simulink model "Robot"  (R2022b)
settings: Solver=FixedStepDiscrete  StartTime=0.0  StopTime=30  FixedStep=0.001  RelTol=1e-3
InitFcn:
  | load("BusConfig.mat");
undefined symbols (not defined in the file or in its folder): DiscIntNeverNeededParam
libraries: slrealtimeethercatlib x119, simulink x20
(part 5 of 7)

== system Robot/Motor1 Torque Control Init Frame/Set MasterState to OP Frame/If Action Subsystem7 ==
  In1 : Inport
  Action Port : ActionPort  ActionPortLabel=if((u1 == 8))
  Discrete-Time Integrator : DiscreteIntegrator  SampleTime=-1  ICPrevOutput=DiscIntNeverNeededParam  ICPrevScaledInput=DiscIntNeverNeededParam
  Out1 : Outport
  wires:
  In1/1 -> Discrete-Time Integrator/1
  Discrete-Time Integrator/1 -> Out1/1

== system Robot/Motor1 Torque Control Init Frame/Set MasterState to SafeOP Frame/If Action Subsystem5 ==
  In1 : Inport
  Action Port : ActionPort  ActionPortLabel=if((u1 > 0.1))
  Out1 : Outport
  wires:
  In1/1 -> Out1/1

== system Robot/Motor1 Torque Control Init Frame/Set MasterState to SafeOP Frame/If Action Subsystem6 ==
  In1 : Inport
  Action Port : ActionPort  ActionPortLabel=else
  Out1 : Outport
  wires:
  In1/1 -> Out1/1

== system Robot/Motor1 Torque Control Init Frame/Set MasterState to SafeOP Frame/If Action Subsystem7 ==
  In1 : Inport
  Action Port : ActionPort  ActionPortLabel=if((u1 == 4))
  Discrete-Time Integrator : DiscreteIntegrator  SampleTime=-1  ICPrevOutput=DiscIntNeverNeededParam  ICPrevScaledInput=DiscIntNeverNeededParam
  Out1 : Outport
  wires:
  In1/1 -> Discrete-Time Integrator/1
  Discrete-Time Integrator/1 -> Out1/1

== system Robot/Motor1 Torque Control Init Frame/State_10_Enable/Subsystem ==
  Case : Inport
  Case Default : Inport  Port=2
  Constant : Constant
  Constant1 : Constant  Value=0
  Constant2 : Constant  Value=TaskIndex
  Merge : Merge
  Switch Case Action Subsystem : Subsystem  TreatAsAtomicUnit=on
  Switch Case Action Subsystem1 : Subsystem  TreatAsAtomicUnit=on
  Enable : Outport
  FinishIndex : Outport  Port=2
  wires:
  Constant/1 -> Switch Case Action Subsystem/1(In1)
  Case/1 -> Switch Case Action Subsystem/Action
  Switch Case Action Subsystem/1(Out1) -> Merge/1
  Merge/1 -> Enable/1
  Case Default/1 -> Switch Case Action Subsystem1/Action
  Constant1/1 -> Switch Case Action Subsystem1/1(In1)
  Switch Case Action Subsystem1/1(Default) -> Merge/2
  Constant2/1 -> FinishIndex/1

== system Robot/Motor1 Torque Control Init Frame/State_11_Enable/Subsystem ==
  Case : Inport
  Case Default : Inport  Port=2
  Constant : Constant
  Constant1 : Constant  Value=0
  Constant2 : Constant  Value=TaskIndex
  Merge : Merge
  Switch Case Action Subsystem : Subsystem  TreatAsAtomicUnit=on
  Switch Case Action Subsystem1 : Subsystem  TreatAsAtomicUnit=on
  Enable : Outport
  FinishIndex : Outport  Port=2
  wires:
  Constant/1 -> Switch Case Action Subsystem/1(In1)
  Case/1 -> Switch Case Action Subsystem/Action
  Switch Case Action Subsystem/1(Out1) -> Merge/1
  Merge/1 -> Enable/1
  Case Default/1 -> Switch Case Action Subsystem1/Action
  Constant1/1 -> Switch Case Action Subsystem1/1(In1)
  Switch Case Action Subsystem1/1(Default) -> Merge/2
  Constant2/1 -> FinishIndex/1

== system Robot/Motor1 Torque Control Init Frame/State_12_Enable/Subsystem ==
  Case : Inport
  Case Default : Inport  Port=2
  Constant : Constant
  Constant1 : Constant  Value=0
  Constant2 : Constant  Value=TaskIndex
  Merge : Merge
  Switch Case Action Subsystem : Subsystem  TreatAsAtomicUnit=on
  Switch Case Action Subsystem1 : Subsystem  TreatAsAtomicUnit=on
  Enable : Outport
  FinishIndex : Outport  Port=2
  wires:
  Constant/1 -> Switch Case Action Subsystem/1(In1)
  Case/1 -> Switch Case Action Subsystem/Action
  Switch Case Action Subsystem/1(Out1) -> Merge/1
  Merge/1 -> Enable/1
  Case Default/1 -> Switch Case Action Subsystem1/Action
  Constant1/1 -> Switch Case Action Subsystem1/1(In1)
  Switch Case Action Subsystem1/1(Default) -> Merge/2
  Constant2/1 -> FinishIndex/1

== system Robot/Motor1 Torque Control Init Frame/State_13_Enable/Subsystem ==
  Case : Inport
  Case Default : Inport  Port=2
  Constant : Constant
  Constant1 : Constant  Value=0
  Constant2 : Constant  Value=TaskIndex
  Merge : Merge
  Switch Case Action Subsystem : Subsystem  TreatAsAtomicUnit=on
  Switch Case Action Subsystem1 : Subsystem  TreatAsAtomicUnit=on
  Enable : Outport
  FinishIndex : Outport  Port=2
  wires:
  Constant/1 -> Switch Case Action Subsystem/1(In1)
  Case/1 -> Switch Case Action Subsystem/Action
  Switch Case Action Subsystem/1(Out1) -> Merge/1
  Merge/1 -> Enable/1
  Case Default/1 -> Switch Case Action Subsystem1/Action
  Constant1/1 -> Switch Case Action Subsystem1/1(In1)
  Switch Case Action Subsystem1/1(Default) -> Merge/2
  Constant2/1 -> FinishIndex/1

== system Robot/Motor1 Torque Control Init Frame/State_1_Enable/Subsystem ==
  Case : Inport
  Case Default : Inport  Port=2
  Constant : Constant
  Constant1 : Constant  Value=0
  Constant2 : Constant  Value=TaskIndex
  Merge : Merge
  Switch Case Action Subsystem : Subsystem  TreatAsAtomicUnit=on
  Switch Case Action Subsystem1 : Subsystem  TreatAsAtomicUnit=on
  Enable : Outport
  FinishIndex : Outport  Port=2
  wires:
  Constant/1 -> Switch Case Action Subsystem/1(In1)
  Case/1 -> Switch Case Action Subsystem/Action
  Switch Case Action Subsystem/1(Out1) -> Merge/1
  Merge/1 -> Enable/1
  Case Default/1 -> Switch Case Action Subsystem1/Action
  Constant1/1 -> Switch Case Action Subsystem1/1(In1)
  Switch Case Action Subsystem1/1(Default) -> Merge/2
  Constant2/1 -> FinishIndex/1

== system Robot/Motor1 Torque Control Init Frame/State_2_Enable/Subsystem ==
  Case : Inport
  Case Default : Inport  Port=2
  Constant : Constant
  Constant1 : Constant  Value=0
  Constant2 : Constant  Value=TaskIndex
  Merge : Merge
  Switch Case Action Subsystem : Subsystem  TreatAsAtomicUnit=on
  Switch Case Action Subsystem1 : Subsystem  TreatAsAtomicUnit=on
  Enable : Outport
  FinishIndex : Outport  Port=2
  wires:
  Constant/1 -> Switch Case Action Subsystem/1(In1)
  Case/1 -> Switch Case Action Subsystem/Action
  Switch Case Action Subsystem/1(Out1) -> Merge/1
  Merge/1 -> Enable/1
  Case Default/1 -> Switch Case Action Subsystem1/Action
  Constant1/1 -> Switch Case Action Subsystem1/1(In1)
  Switch Case Action Subsystem1/1(Default) -> Merge/2
  Constant2/1 -> FinishIndex/1

== system Robot/Motor1 Torque Control Init Frame/State_3_Enable/Subsystem ==
  Case : Inport
  Case Default : Inport  Port=2
  Constant : Constant
  Constant1 : Constant  Value=0
  Constant2 : Constant  Value=TaskIndex
  Merge : Merge
  Switch Case Action Subsystem : Subsystem  TreatAsAtomicUnit=on
  Switch Case Action Subsystem1 : Subsystem  TreatAsAtomicUnit=on
  Enable : Outport
  FinishIndex : Outport  Port=2
  wires:
  Constant/1 -> Switch Case Action Subsystem/1(In1)
  Case/1 -> Switch Case Action Subsystem/Action
  Switch Case Action Subsystem/1(Out1) -> Merge/1
  Merge/1 -> Enable/1
  Case Default/1 -> Switch Case Action Subsystem1/Action
  Constant1/1 -> Switch Case Action Subsystem1/1(In1)
  Switch Case Action Subsystem1/1(Default) -> Merge/2
  Constant2/1 -> FinishIndex/1

== system Robot/Motor1 Torque Control Init Frame/State_4_Enable/Subsystem ==
  Case : Inport
  Case Default : Inport  Port=2
  Constant : Constant
  Constant1 : Constant  Value=0
  Constant2 : Constant  Value=TaskIndex
  Merge : Merge
  Switch Case Action Subsystem : Subsystem  TreatAsAtomicUnit=on
  Switch Case Action Subsystem1 : Subsystem  TreatAsAtomicUnit=on
  Enable : Outport
  FinishIndex : Outport  Port=2
  wires:
  Constant/1 -> Switch Case Action Subsystem/1(In1)
  Case/1 -> Switch Case Action Subsystem/Action
  Switch Case Action Subsystem/1(Out1) -> Merge/1
  Merge/1 -> Enable/1
  Case Default/1 -> Switch Case Action Subsystem1/Action
  Constant1/1 -> Switch Case Action Subsystem1/1(In1)
  Switch Case Action Subsystem1/1(Default) -> Merge/2
  Constant2/1 -> FinishIndex/1

== system Robot/Motor1 Torque Control Init Frame/State_5_Enable/Subsystem ==
  Case : Inport
  Case Default : Inport  Port=2
  Constant : Constant
  Constant1 : Constant  Value=0
  Constant2 : Constant  Value=TaskIndex
  Merge : Merge
  Switch Case Action Subsystem : Subsystem  TreatAsAtomicUnit=on
  Switch Case Action Subsystem1 : Subsystem  TreatAsAtomicUnit=on
  Enable : Outport
  FinishIndex : Outport  Port=2
  wires:
  Constant/1 -> Switch Case Action Subsystem/1(In1)
  Case/1 -> Switch Case Action Subsystem/Action
  Switch Case Action Subsystem/1(Out1) -> Merge/1
  Merge/1 -> Enable/1
  Case Default/1 -> Switch Case Action Subsystem1/Action
  Constant1/1 -> Switch Case Action Subsystem1/1(In1)
  Switch Case Action Subsystem1/1(Default) -> Merge/2
  Constant2/1 -> FinishIndex/1

== system Robot/Motor1 Torque Control Init Frame/State_6_Enable/Subsystem ==
  Case : Inport
  Case Default : Inport  Port=2
  Constant : Constant
  Constant1 : Constant  Value=0
  Constant2 : Constant  Value=TaskIndex
  Merge : Merge
  Switch Case Action Subsystem : Subsystem  TreatAsAtomicUnit=on
  Switch Case Action Subsystem1 : Subsystem  TreatAsAtomicUnit=on
  Enable : Outport
  FinishIndex : Outport  Port=2
  wires:
  Constant/1 -> Switch Case Action Subsystem/1(In1)
  Case/1 -> Switch Case Action Subsystem/Action
  Switch Case Action Subsystem/1(Out1) -> Merge/1
  Merge/1 -> Enable/1
  Case Default/1 -> Switch Case Action Subsystem1/Action
  Constant1/1 -> Switch Case Action Subsystem1/1(In1)
  Switch Case Action Subsystem1/1(Default) -> Merge/2
  Constant2/1 -> FinishIndex/1

== system Robot/Motor1 Torque Control Init Frame/State_7_Enable/Subsystem ==
  Case : Inport
  Case Default : Inport  Port=2
  Constant : Constant
  Constant1 : Constant  Value=0
  Constant2 : Constant  Value=TaskIndex
  Merge : Merge
  Switch Case Action Subsystem : Subsystem  TreatAsAtomicUnit=on
  Switch Case Action Subsystem1 : Subsystem  TreatAsAtomicUnit=on
  Enable : Outport
  FinishIndex : Outport  Port=2
  wires:
  Constant/1 -> Switch Case Action Subsystem/1(In1)
  Case/1 -> Switch Case Action Subsystem/Action
  Switch Case Action Subsystem/1(Out1) -> Merge/1
  Merge/1 -> Enable/1
  Case Default/1 -> Switch Case Action Subsystem1/Action
  Constant1/1 -> Switch Case Action Subsystem1/1(In1)
  Switch Case Action Subsystem1/1(Default) -> Merge/2
  Constant2/1 -> FinishIndex/1

== system Robot/Motor1 Torque Control Init Frame/State_8_Enable/Subsystem ==
  Case : Inport
  Case Default : Inport  Port=2
  Constant : Constant
  Constant1 : Constant  Value=0
  Constant2 : Constant  Value=TaskIndex
  Merge : Merge
  Switch Case Action Subsystem : Subsystem  TreatAsAtomicUnit=on
  Switch Case Action Subsystem1 : Subsystem  TreatAsAtomicUnit=on
  Enable : Outport
  FinishIndex : Outport  Port=2
  wires:
  Constant/1 -> Switch Case Action Subsystem/1(In1)
  Case/1 -> Switch Case Action Subsystem/Action
  Switch Case Action Subsystem/1(Out1) -> Merge/1
  Merge/1 -> Enable/1
  Case Default/1 -> Switch Case Action Subsystem1/Action
  Constant1/1 -> Switch Case Action Subsystem1/1(In1)
  Switch Case Action Subsystem1/1(Default) -> Merge/2
  Constant2/1 -> FinishIndex/1

== system Robot/Motor1 Torque Control Init Frame/State_9_Enable/Subsystem ==
  Case : Inport
  Case Default : Inport  Port=2
  Constant : Constant
  Constant1 : Constant  Value=0
  Constant2 : Constant  Value=TaskIndex
  Merge : Merge
  Switch Case Action Subsystem : Subsystem  TreatAsAtomicUnit=on
  Switch Case Action Subsystem1 : Subsystem  TreatAsAtomicUnit=on
  Enable : Outport
  FinishIndex : Outport  Port=2
  wires:
  Constant/1 -> Switch Case Action Subsystem/1(In1)
  Case/1 -> Switch Case Action Subsystem/Action
  Switch Case Action Subsystem/1(Out1) -> Merge/1
  Merge/1 -> Enable/1
  Case Default/1 -> Switch Case Action Subsystem1/Action
  Constant1/1 -> Switch Case Action Subsystem1/1(In1)
  Switch Case Action Subsystem1/1(Default) -> Merge/2
  Constant2/1 -> FinishIndex/1

== system Robot/Motor2 Torque Control Init Frame/Get MasterState OP Frame/If Action Subsystem5 ==
  In1 : Inport
  Action Port : ActionPort  ActionPortLabel=if((u1 == 8))
  Out1 : Outport
  wires:
  In1/1 -> Out1/1

== system Robot/Motor2 Torque Control Init Frame/Get MasterState OP Frame/If Action Subsystem6 ==
  In1 : Inport
  Action Port : ActionPort  ActionPortLabel=else
  Out1 : Outport
  wires:
  In1/1 -> Out1/1

== system Robot/Motor2 Torque Control Init Frame/Get MasterState OP Frame/If Action Subsystem7 ==
  In1 : Inport
  Action Port : ActionPort  ActionPortLabel=if((u1 == 4663))
  Discrete-Time Integrator : DiscreteIntegrator  SampleTime=-1  ICPrevOutput=DiscIntNeverNeededParam  ICPrevScaledInput=DiscIntNeverNeededParam
  Out1 : Outport
  wires:
  In1/1 -> Discrete-Time Integrator/1
  Discrete-Time Integrator/1 -> Out1/1

== system Robot/Motor2 Torque Control Init Frame/PDO Set 0x6040:6->7->15 Frame/If Action Subsystem ==
  In1 : Inport
  Action Port : ActionPort  ActionPortLabel=if((u1 == 720)&(u2 == 500))
  Out1 : Outport
  wires:
  In1/1 -> Out1/1

== system Robot/Motor2 Torque Control Init Frame/PDO Set 0x6040:6->7->15 Frame/If Action Subsystem1 ==
  In1 : Inport
  Action Port : ActionPort  ActionPortLabel=elseif((u1 == 689)&(u2 == 500))
  Out1 : Outport
  wires:
  In1/1 -> Out1/1

== system Robot/Motor2 Torque Control Init Frame/PDO Set 0x6040:6->7->15 Frame/If Action Subsystem2 ==
  In1 : Inport
  Action Port : ActionPort  ActionPortLabel=elseif( (u1 == 691)&(u2 == 500))
  Out1 : Outport
  wires:
  In1/1 -> Out1/1

== system Robot/Motor2 Torque Control Init Frame/PDO Set 0x6040:6->7->15 Frame/If Action Subsystem4 ==
  In1 : Inport
  Action Port : ActionPort  ActionPortLabel=else
  Out1 : Outport
  wires:
  In1/1 -> Out1/1

== system Robot/Motor2 Torque Control Init Frame/PDO Set 0x6040:6->7->15 Frame/If Action Subsystem5 ==
  In1 : Inport
  Action Port : ActionPort  ActionPortLabel=if((u1 >= 0.1))
  Out1 : Outport
  wires:
  In1/1 -> Out1/1

== system Robot/Motor2 Torque Control Init Frame/PDO Set 0x6040:6->7->15 Frame/If Action Subsystem6 ==
  In1 : Inport
  Action Port : ActionPort  ActionPortLabel=else
  Out1 : Outport
  wires:
  In1/1 -> Out1/1

== system Robot/Motor2 Torque Control Init Frame/PDO Set 0x6040:6->7->15 Frame/If Action Subsystem7 ==
  In1 : Inport
  Action Port : ActionPort  ActionPortLabel=if((u1 == 4663)|(u1 == 4791))
  Discrete-Time Integrator : DiscreteIntegrator  SampleTime=-1  ICPrevOutput=DiscIntNeverNeededParam  ICPrevScaledInput=DiscIntNeverNeededParam
  Out1 : Outport
  wires:
  In1/1 -> Discrete-Time Integrator/1
  Discrete-Time Integrator/1 -> Out1/1

== system Robot/Motor2 Torque Control Init Frame/SDO Get 0x6075 Frame/If Action Subsystem5 ==
  In1 : Inport
  Action Port : ActionPort  ActionPortLabel=if((u1 == 2))
  Out1 : Outport
  wires:
  In1/1 -> Out1/1

== system Robot/Motor2 Torque Control Init Frame/SDO Get 0x6075 Frame/If Action Subsystem6 ==
  In1 : Inport
  Action Port : ActionPort  ActionPortLabel=else
  Out1 : Outport
  wires:
  In1/1 -> Out1/1

== system Robot/Motor2 Torque Control Init Frame/SDO Get 0x6075 Frame/If Action Subsystem7 ==
  In1 : Inport
  Action Port : ActionPort  ActionPortLabel=if((u1 == 4663))
  Discrete-Time Integrator : DiscreteIntegrator  SampleTime=-1  ICPrevOutput=DiscIntNeverNeededParam  ICPrevScaledInput=DiscIntNeverNeededParam
  Out1 : Outport
  wires:
  In1/1 -> Discrete-Time Integrator/1
  Discrete-Time Integrator/1 -> Out1/1

== system Robot/Motor2 Torque Control Init Frame/SDO Set 0x6040:15 Frame/If Action Subsystem1 ==
  In1 : Inport
  Action Port : ActionPort  ActionPortLabel=if((u1 >= 0.1))
  Out1 : Outport
  wires:
  In1/1 -> Out1/1

== system Robot/Motor2 Torque Control Init Frame/SDO Set 0x6040:15 Frame/If Action Subsystem2 ==
  In1 : Inport
  Action Port : ActionPort  ActionPortLabel=else
  Out1 : Outport
  wires:
  In1/1 -> Out1/1

== system Robot/Motor2 Torque Control Init Frame/SDO Set 0x6040:15 Frame/If Action Subsystem3 ==
  In1 : Inport
  Action Port : ActionPort  ActionPortLabel=if((u1 == u2))
  Discrete-Time Integrator : DiscreteIntegrator  SampleTime=-1  ICPrevOutput=DiscIntNeverNeededParam  ICPrevScaledInput=DiscIntNeverNeededParam
  Out1 : Outport
  wires:
  In1/1 -> Discrete-Time Integrator/1
  Discrete-Time Integrator/1 -> Out1/1

== system Robot/Motor2 Torque Control Init Frame/SDO Set 0x6040:15 Frame/If Action Subsystem5 ==
  In1 : Inport
  Action Port : ActionPort  ActionPortLabel=if((u1 == 2))
  Out1 : Outport
  wires:
  In1/1 -> Out1/1

== system Robot/Motor2 Torque Control Init Frame/SDO Set 0x6040:15 Frame/If Action Subsystem6 ==
  In1 : Inport
  Action Port : ActionPort  ActionPortLabel=else
  Out1 : Outport
  wires:
  In1/1 -> Out1/1

== system Robot/Motor2 Torque Control Init Frame/SDO Set 0x6040:15 Frame/If Action Subsystem7 ==
  In1 : Inport
  Action Port : ActionPort  ActionPortLabel=if((u1 == 4663))
  Discrete-Time Integrator : DiscreteIntegrator  SampleTime=-1  ICPrevOutput=DiscIntNeverNeededParam  ICPrevScaledInput=DiscIntNeverNeededParam
  Out1 : Outport
  wires:
  In1/1 -> Discrete-Time Integrator/1
  Discrete-Time Integrator/1 -> Out1/1

== system Robot/Motor2 Torque Control Init Frame/SDO Set 0x6040:31 Frame/If Action Subsystem1 ==
  In1 : Inport
  Action Port : ActionPort  ActionPortLabel=if((u1 >= 0.1))
  Out1 : Outport
  wires:
  In1/1 -> Out1/1

== system Robot/Motor2 Torque Control Init Frame/SDO Set 0x6040:31 Frame/If Action Subsystem2 ==
  In1 : Inport
  Action Port : ActionPort  ActionPortLabel=else
  Out1 : Outport
  wires:
  In1/1 -> Out1/1

== system Robot/Motor2 Torque Control Init Frame/SDO Set 0x6040:31 Frame/If Action Subsystem3 ==
  In1 : Inport
  Action Port : ActionPort  ActionPortLabel=if((u1 == u2))
  Discrete-Time Integrator : DiscreteIntegrator  SampleTime=-1  ICPrevOutput=DiscIntNeverNeededParam  ICPrevScaledInput=DiscIntNeverNeededParam
  Out1 : Outport
  wires:
  In1/1 -> Discrete-Time Integrator/1
  Discrete-Time Integrator/1 -> Out1/1

== system Robot/Motor2 Torque Control Init Frame/SDO Set 0x6040:31 Frame/If Action Subsystem5 ==
  In1 : Inport
  Action Port : ActionPort  ActionPortLabel=if((u1 == 2))
  Out1 : Outport
  wires:
  In1/1 -> Out1/1

== system Robot/Motor2 Torque Control Init Frame/SDO Set 0x6040:31 Frame/If Action Subsystem6 ==
  In1 : Inport
  Action Port : ActionPort  ActionPortLabel=else
  Out1 : Outport
  wires:
  In1/1 -> Out1/1

== system Robot/Motor2 Torque Control Init Frame/SDO Set 0x6040:31 Frame/If Action Subsystem7 ==
  In1 : Inport
  Action Port : ActionPort  ActionPortLabel=if((u1 == 4663))
  Discrete-Time Integrator : DiscreteIntegrator  SampleTime=-1  ICPrevOutput=DiscIntNeverNeededParam  ICPrevScaledInput=DiscIntNeverNeededParam
  Out1 : Outport
  wires:
  In1/1 -> Discrete-Time Integrator/1
  Discrete-Time Integrator/1 -> Out1/1

== system Robot/Motor2 Torque Control Init Frame/SDO Set 0x6040:6 Frame/If Action Subsystem1 ==
  In1 : Inport
  Action Port : ActionPort  ActionPortLabel=if((u1 >= 0.1))
  Out1 : Outport
  wires:
  In1/1 -> Out1/1

== system Robot/Motor2 Torque Control Init Frame/SDO Set 0x6040:6 Frame/If Action Subsystem2 ==
  In1 : Inport
  Action Port : ActionPort  ActionPortLabel=else
  Out1 : Outport
  wires:
  In1/1 -> Out1/1

== system Robot/Motor2 Torque Control Init Frame/SDO Set 0x6040:6 Frame/If Action Subsystem3 ==
  In1 : Inport
  Action Port : ActionPort  ActionPortLabel=if((u1 == u2))
  Discrete-Time Integrator : DiscreteIntegrator  SampleTime=-1  ICPrevOutput=DiscIntNeverNeededParam  ICPrevScaledInput=DiscIntNeverNeededParam
  Out1 : Outport
  wires:
  In1/1 -> Discrete-Time Integrator/1
  Discrete-Time Integrator/1 -> Out1/1

== system Robot/Motor2 Torque Control Init Frame/SDO Set 0x6040:6 Frame/If Action Subsystem5 ==
  In1 : Inport
  Action Port : ActionPort  ActionPortLabel=if((u1 == 2))
  Out1 : Outport
  wires:
  In1/1 -> Out1/1

== system Robot/Motor2 Torque Control Init Frame/SDO Set 0x6040:6 Frame/If Action Subsystem6 ==
  In1 : Inport
  Action Port : ActionPort  ActionPortLabel=else
  Out1 : Outport
  wires:
  In1/1 -> Out1/1

== system Robot/Motor2 Torque Control Init Frame/SDO Set 0x6040:6 Frame/If Action Subsystem7 ==
  In1 : Inport
  Action Port : ActionPort  ActionPortLabel=if((u1 == 4663))
  Discrete-Time Integrator : DiscreteIntegrator  SampleTime=-1  ICPrevOutput=DiscIntNeverNeededParam  ICPrevScaledInput=DiscIntNeverNeededParam
  Out1 : Outport
  wires:
  In1/1 -> Discrete-Time Integrator/1
  Discrete-Time Integrator/1 -> Out1/1

== system Robot/Motor2 Torque Control Init Frame/SDO Set 0x6040:7 Frame/If Action Subsystem1 ==
  In1 : Inport
  Action Port : ActionPort  ActionPortLabel=if((u1 >= 0.1))
  Out1 : Outport
  wires:
  In1/1 -> Out1/1

== system Robot/Motor2 Torque Control Init Frame/SDO Set 0x6040:7 Frame/If Action Subsystem2 ==
  In1 : Inport
  Action Port : ActionPort  ActionPortLabel=else
  Out1 : Outport
  wires:
  In1/1 -> Out1/1

== system Robot/Motor2 Torque Control Init Frame/SDO Set 0x6040:7 Frame/If Action Subsystem3 ==
  In1 : Inport
  Action Port : ActionPort  ActionPortLabel=if((u1 == u2))
  Discrete-Time Integrator : DiscreteIntegrator  SampleTime=-1  ICPrevOutput=DiscIntNeverNeededParam  ICPrevScaledInput=DiscIntNeverNeededParam
  Out1 : Outport
  wires:
  In1/1 -> Discrete-Time Integrator/1
  Discrete-Time Integrator/1 -> Out1/1

== system Robot/Motor2 Torque Control Init Frame/SDO Set 0x6040:7 Frame/If Action Subsystem5 ==
  In1 : Inport
  Action Port : ActionPort  ActionPortLabel=if((u1 == 2))
  Out1 : Outport
  wires:
  In1/1 -> Out1/1

== system Robot/Motor2 Torque Control Init Frame/SDO Set 0x6040:7 Frame/If Action Subsystem6 ==
  In1 : Inport
  Action Port : ActionPort  ActionPortLabel=else
  Out1 : Outport
  wires:
  In1/1 -> Out1/1

== system Robot/Motor2 Torque Control Init Frame/SDO Set 0x6040:7 Frame/If Action Subsystem7 ==
  In1 : Inport
  Action Port : ActionPort  ActionPortLabel=if((u1 == 4663))
  Discrete-Time Integrator : DiscreteIntegrator  SampleTime=-1  ICPrevOutput=DiscIntNeverNeededParam  ICPrevScaledInput=DiscIntNeverNeededParam
  Out1 : Outport
  wires:
  In1/1 -> Discrete-Time Integrator/1
  Discrete-Time Integrator/1 -> Out1/1

== system Robot/Motor2 Torque Control Init Frame/SDO Set 0x6060:10 Frame/If Action Subsystem5 ==
  In1 : Inport
  Action Port : ActionPort  ActionPortLabel=if((u1 == 2))
  Out1 : Outport
  wires:
  In1/1 -> Out1/1

== system Robot/Motor2 Torque Control Init Frame/SDO Set 0x6060:10 Frame/If Action Subsystem6 ==
  In1 : Inport
  Action Port : ActionPort  ActionPortLabel=else
  Out1 : Outport
  wires:
  In1/1 -> Out1/1

== system Robot/Motor2 Torque Control Init Frame/SDO Set 0x6060:10 Frame/If Action Subsystem7 ==
  In1 : Inport
  Action Port : ActionPort  ActionPortLabel=if((u1 == 4663))
  Discrete-Time Integrator : DiscreteIntegrator  SampleTime=-1  ICPrevOutput=DiscIntNeverNeededParam  ICPrevScaledInput=DiscIntNeverNeededParam
  Out1 : Outport
  wires:
  In1/1 -> Discrete-Time Integrator/1
  Discrete-Time Integrator/1 -> Out1/1

== system Robot/Motor2 Torque Control Init Frame/SDO Set 0x6060:6 Frame/If Action Subsystem5 ==
  In1 : Inport
  Action Port : ActionPort  ActionPortLabel=if((u1 == 2))
  Out1 : Outport
  wires:
  In1/1 -> Out1/1

== system Robot/Motor2 Torque Control Init Frame/SDO Set 0x6060:6 Frame/If Action Subsystem6 ==
  In1 : Inport
  Action Port : ActionPort  ActionPortLabel=else
  Out1 : Outport
  wires:
  In1/1 -> Out1/1

== system Robot/Motor2 Torque Control Init Frame/SDO Set 0x6060:6 Frame/If Action Subsystem7 ==
  In1 : Inport
  Action Port : ActionPort  ActionPortLabel=if((u1 == 4663))
  Discrete-Time Integrator : DiscreteIntegrator  SampleTime=-1  ICPrevOutput=DiscIntNeverNeededParam  ICPrevScaledInput=DiscIntNeverNeededParam
  Out1 : Outport
  wires:
  In1/1 -> Discrete-Time Integrator/1
  Discrete-Time Integrator/1 -> Out1/1

== system Robot/Motor2 Torque Control Init Frame/SDO Set 0x6080:-1 Frame/If Action Subsystem5 ==
  In1 : Inport
  Action Port : ActionPort  ActionPortLabel=if((u1 == 2))
  Out1 : Outport
  wires:
  In1/1 -> Out1/1

== system Robot/Motor2 Torque Control Init Frame/SDO Set 0x6080:-1 Frame/If Action Subsystem6 ==
  In1 : Inport
  Action Port : ActionPort  ActionPortLabel=else
  Out1 : Outport
  wires:
  In1/1 -> Out1/1

== system Robot/Motor2 Torque Control Init Frame/SDO Set 0x6080:-1 Frame/If Action Subsystem7 ==
  In1 : Inport
  Action Port : ActionPort  ActionPortLabel=if((u1 == 4663))
  Discrete-Time Integrator : DiscreteIntegrator  SampleTime=-1  ICPrevOutput=DiscIntNeverNeededParam  ICPrevScaledInput=DiscIntNeverNeededParam
  Out1 : Outport
  wires:
  In1/1 -> Discrete-Time Integrator/1
  Discrete-Time Integrator/1 -> Out1/1

== system Robot/Motor2 Torque Control Init Frame/SDO Set 0x6098:35 Frame/If Action Subsystem5 ==
  In1 : Inport
  Action Port : ActionPort  ActionPortLabel=if((u1 == 2))
  Out1 : Outport
  wires:
  In1/1 -> Out1/1

== system Robot/Motor2 Torque Control Init Frame/SDO Set 0x6098:35 Frame/If Action Subsystem6 ==
  In1 : Inport
  Action Port : ActionPort  ActionPortLabel=else
  Out1 : Outport
  wires:
  In1/1 -> Out1/1

== system Robot/Motor2 Torque Control Init Frame/SDO Set 0x6098:35 Frame/If Action Subsystem7 ==
  In1 : Inport
  Action Port : ActionPort  ActionPortLabel=if((u1 == 4663))
  Discrete-Time Integrator : DiscreteIntegrator  SampleTime=-1  ICPrevOutput=DiscIntNeverNeededParam  ICPrevScaledInput=DiscIntNeverNeededParam
  Out1 : Outport
  wires:
  In1/1 -> Discrete-Time Integrator/1
  Discrete-Time Integrator/1 -> Out1/1

== system Robot/Motor2 Torque Control Init Frame/Set MasterState to OP Frame/If Action Subsystem5 ==
  In1 : Inport
  Action Port : ActionPort  ActionPortLabel=if((u1 > 0.1))
  Out1 : Outport
  wires:
  In1/1 -> Out1/1

== system Robot/Motor2 Torque Control Init Frame/Set MasterState to OP Frame/If Action Subsystem6 ==
  In1 : Inport
  Action Port : ActionPort  ActionPortLabel=else
  Out1 : Outport
  wires:
  In1/1 -> Out1/1

== system Robot/Motor2 Torque Control Init Frame/Set MasterState to OP Frame/If Action Subsystem7 ==
  In1 : Inport
  Action Port : ActionPort  ActionPortLabel=if((u1 == 8))
  Discrete-Time Integrator : DiscreteIntegrator  SampleTime=-1  ICPrevOutput=DiscIntNeverNeededParam  ICPrevScaledInput=DiscIntNeverNeededParam
  Out1 : Outport
  wires:
  In1/1 -> Discrete-Time Integrator/1
  Discrete-Time Integrator/1 -> Out1/1

== system Robot/Motor2 Torque Control Init Frame/Set MasterState to SafeOP Frame/If Action Subsystem5 ==
  In1 : Inport
  Action Port : ActionPort  ActionPortLabel=if((u1 > 0.1))
  Out1 : Outport
  wires:
  In1/1 -> Out1/1

== system Robot/Motor2 Torque Control Init Frame/Set MasterState to SafeOP Frame/If Action Subsystem6 ==
  In1 : Inport
  Action Port : ActionPort  ActionPortLabel=else
  Out1 : Outport
  wires:
  In1/1 -> Out1/1

== system Robot/Motor2 Torque Control Init Frame/Set MasterState to SafeOP Frame/If Action Subsystem7 ==
  In1 : Inport
  Action Port : ActionPort  ActionPortLabel=if((u1 == 4))
  Discrete-Time Integrator : DiscreteIntegrator  SampleTime=-1  ICPrevOutput=DiscIntNeverNeededParam  ICPrevScaledInput=DiscIntNeverNeededParam
  Out1 : Outport
  wires:
  In1/1 -> Discrete-Time Integrator/1
  Discrete-Time Integrator/1 -> Out1/1

== system Robot/Motor2 Torque Control Init Frame/State_10_Enable/Subsystem ==
  Case : Inport
  Case Default : Inport  Port=2
  Constant : Constant
  Constant1 : Constant  Value=0
  Constant2 : Constant  Value=TaskIndex
  Merge : Merge
  Switch Case Action Subsystem : Subsystem  TreatAsAtomicUnit=on
  Switch Case Action Subsystem1 : Subsystem  TreatAsAtomicUnit=on
  Enable : Outport
  FinishIndex : Outport  Port=2
  wires:
  Constant/1 -> Switch Case Action Subsystem/1(In1)
  Case/1 -> Switch Case Action Subsystem/Action
  Switch Case Action Subsystem/1(Out1) -> Merge/1
  Merge/1 -> Enable/1
  Case Default/1 -> Switch Case Action Subsystem1/Action
  Constant1/1 -> Switch Case Action Subsystem1/1(In1)
  Switch Case Action Subsystem1/1(Default) -> Merge/2
  Constant2/1 -> FinishIndex/1

== system Robot/Motor2 Torque Control Init Frame/State_11_Enable/Subsystem ==
  Case : Inport
  Case Default : Inport  Port=2
  Constant : Constant
  Constant1 : Constant  Value=0
  Constant2 : Constant  Value=TaskIndex
  Merge : Merge
  Switch Case Action Subsystem : Subsystem  TreatAsAtomicUnit=on
  Switch Case Action Subsystem1 : Subsystem  TreatAsAtomicUnit=on
  Enable : Outport
  FinishIndex : Outport  Port=2
  wires:
  Constant/1 -> Switch Case Action Subsystem/1(In1)
  Case/1 -> Switch Case Action Subsystem/Action
  Switch Case Action Subsystem/1(Out1) -> Merge/1
  Merge/1 -> Enable/1
  Case Default/1 -> Switch Case Action Subsystem1/Action
  Constant1/1 -> Switch Case Action Subsystem1/1(In1)
  Switch Case Action Subsystem1/1(Default) -> Merge/2
  Constant2/1 -> FinishIndex/1

== system Robot/Motor2 Torque Control Init Frame/State_12_Enable/Subsystem ==
  Case : Inport
  Case Default : Inport  Port=2
  Constant : Constant
  Constant1 : Constant  Value=0
  Constant2 : Constant  Value=TaskIndex
  Merge : Merge
  Switch Case Action Subsystem : Subsystem  TreatAsAtomicUnit=on
  Switch Case Action Subsystem1 : Subsystem  TreatAsAtomicUnit=on
  Enable : Outport
  FinishIndex : Outport  Port=2
  wires:
  Constant/1 -> Switch Case Action Subsystem/1(In1)
  Case/1 -> Switch Case Action Subsystem/Action
  Switch Case Action Subsystem/1(Out1) -> Merge/1
  Merge/1 -> Enable/1
  Case Default/1 -> Switch Case Action Subsystem1/Action
  Constant1/1 -> Switch Case Action Subsystem1/1(In1)
  Switch Case Action Subsystem1/1(Default) -> Merge/2
  Constant2/1 -> FinishIndex/1

== system Robot/Motor2 Torque Control Init Frame/State_13_Enable/Subsystem ==
  Case : Inport
  Case Default : Inport  Port=2
  Constant : Constant
  Constant1 : Constant  Value=0
  Constant2 : Constant  Value=TaskIndex
  Merge : Merge
  Switch Case Action Subsystem : Subsystem  TreatAsAtomicUnit=on
  Switch Case Action Subsystem1 : Subsystem  TreatAsAtomicUnit=on
  Enable : Outport
  FinishIndex : Outport  Port=2
  wires:
  Constant/1 -> Switch Case Action Subsystem/1(In1)
  Case/1 -> Switch Case Action Subsystem/Action
  Switch Case Action Subsystem/1(Out1) -> Merge/1
  Merge/1 -> Enable/1
  Case Default/1 -> Switch Case Action Subsystem1/Action
  Constant1/1 -> Switch Case Action Subsystem1/1(In1)
  Switch Case Action Subsystem1/1(Default) -> Merge/2
  Constant2/1 -> FinishIndex/1

== system Robot/Motor2 Torque Control Init Frame/State_1_Enable/Subsystem ==
  Case : Inport
  Case Default : Inport  Port=2
  Constant : Constant
  Constant1 : Constant  Value=0
  Constant2 : Constant  Value=TaskIndex
  Merge : Merge
  Switch Case Action Subsystem : Subsystem  TreatAsAtomicUnit=on
  Switch Case Action Subsystem1 : Subsystem  TreatAsAtomicUnit=on
  Enable : Outport
  FinishIndex : Outport  Port=2
  wires:
  Constant/1 -> Switch Case Action Subsystem/1(In1)
  Case/1 -> Switch Case Action Subsystem/Action
  Switch Case Action Subsystem/1(Out1) -> Merge/1
  Merge/1 -> Enable/1
  Case Default/1 -> Switch Case Action Subsystem1/Action
  Constant1/1 -> Switch Case Action Subsystem1/1(In1)
  Switch Case Action Subsystem1/1(Default) -> Merge/2
  Constant2/1 -> FinishIndex/1

== system Robot/Motor2 Torque Control Init Frame/State_2_Enable/Subsystem ==
  Case : Inport
  Case Default : Inport  Port=2
  Constant : Constant
  Constant1 : Constant  Value=0
  Constant2 : Constant  Value=TaskIndex
  Merge : Merge
  Switch Case Action Subsystem : Subsystem  TreatAsAtomicUnit=on
  Switch Case Action Subsystem1 : Subsystem  TreatAsAtomicUnit=on
  Enable : Outport
  FinishIndex : Outport  Port=2
  wires:
  Constant/1 -> Switch Case Action Subsystem/1(In1)
  Case/1 -> Switch Case Action Subsystem/Action
  Switch Case Action Subsystem/1(Out1) -> Merge/1
  Merge/1 -> Enable/1
  Case Default/1 -> Switch Case Action Subsystem1/Action
  Constant1/1 -> Switch Case Action Subsystem1/1(In1)
  Switch Case Action Subsystem1/1(Default) -> Merge/2
  Constant2/1 -> FinishIndex/1

== system Robot/Motor2 Torque Control Init Frame/State_3_Enable/Subsystem ==
  Case : Inport
  Case Default : Inport  Port=2
  Constant : Constant
  Constant1 : Constant  Value=0
  Constant2 : Constant  Value=TaskIndex
  Merge : Merge
  Switch Case Action Subsystem : Subsystem  TreatAsAtomicUnit=on
  Switch Case Action Subsystem1 : Subsystem  TreatAsAtomicUnit=on
  Enable : Outport
  FinishIndex : Outport  Port=2
  wires:
  Constant/1 -> Switch Case Action Subsystem/1(In1)
  Case/1 -> Switch Case Action Subsystem/Action
  Switch Case Action Subsystem/1(Out1) -> Merge/1
  Merge/1 -> Enable/1
  Case Default/1 -> Switch Case Action Subsystem1/Action
  Constant1/1 -> Switch Case Action Subsystem1/1(In1)
  Switch Case Action Subsystem1/1(Default) -> Merge/2
  Constant2/1 -> FinishIndex/1

== system Robot/Motor2 Torque Control Init Frame/State_4_Enable/Subsystem ==
  Case : Inport
  Case Default : Inport  Port=2
  Constant : Constant
  Constant1 : Constant  Value=0
  Constant2 : Constant  Value=TaskIndex
  Merge : Merge
  Switch Case Action Subsystem : Subsystem  TreatAsAtomicUnit=on
  Switch Case Action Subsystem1 : Subsystem  TreatAsAtomicUnit=on
  Enable : Outport
  FinishIndex : Outport  Port=2
  wires:
  Constant/1 -> Switch Case Action Subsystem/1(In1)
  Case/1 -> Switch Case Action Subsystem/Action
  Switch Case Action Subsystem/1(Out1) -> Merge/1
  Merge/1 -> Enable/1
  Case Default/1 -> Switch Case Action Subsystem1/Action
  Constant1/1 -> Switch Case Action Subsystem1/1(In1)
  Switch Case Action Subsystem1/1(Default) -> Merge/2
  Constant2/1 -> FinishIndex/1

== system Robot/Motor2 Torque Control Init Frame/State_5_Enable/Subsystem ==
  Case : Inport
  Case Default : Inport  Port=2
  Constant : Constant
  Constant1 : Constant  Value=0
  Constant2 : Constant  Value=TaskIndex
  Merge : Merge
  Switch Case Action Subsystem : Subsystem  TreatAsAtomicUnit=on
  Switch Case Action Subsystem1 : Subsystem  TreatAsAtomicUnit=on
  Enable : Outport
  FinishIndex : Outport  Port=2
  wires:
  Constant/1 -> Switch Case Action Subsystem/1(In1)
  Case/1 -> Switch Case Action Subsystem/Action
  Switch Case Action Subsystem/1(Out1) -> Merge/1
  Merge/1 -> Enable/1
  Case Default/1 -> Switch Case Action Subsystem1/Action
  Constant1/1 -> Switch Case Action Subsystem1/1(In1)
  Switch Case Action Subsystem1/1(Default) -> Merge/2
  Constant2/1 -> FinishIndex/1

== system Robot/Motor2 Torque Control Init Frame/State_6_Enable/Subsystem ==
  Case : Inport
  Case Default : Inport  Port=2
  Constant : Constant
  Constant1 : Constant  Value=0
  Constant2 : Constant  Value=TaskIndex
  Merge : Merge
  Switch Case Action Subsystem : Subsystem  TreatAsAtomicUnit=on
  Switch Case Action Subsystem1 : Subsystem  TreatAsAtomicUnit=on
  Enable : Outport
  FinishIndex : Outport  Port=2
  wires:
  Constant/1 -> Switch Case Action Subsystem/1(In1)
  Case/1 -> Switch Case Action Subsystem/Action
  Switch Case Action Subsystem/1(Out1) -> Merge/1
  Merge/1 -> Enable/1
  Case Default/1 -> Switch Case Action Subsystem1/Action
  Constant1/1 -> Switch Case Action Subsystem1/1(In1)
  Switch Case Action Subsystem1/1(Default) -> Merge/2
  Constant2/1 -> FinishIndex/1

== system Robot/Motor2 Torque Control Init Frame/State_7_Enable/Subsystem ==
  Case : Inport
  Case Default : Inport  Port=2
  Constant : Constant
  Constant1 : Constant  Value=0
  Constant2 : Constant  Value=TaskIndex
  Merge : Merge
  Switch Case Action Subsystem : Subsystem  TreatAsAtomicUnit=on
  Switch Case Action Subsystem1 : Subsystem  TreatAsAtomicUnit=on
  Enable : Outport
  FinishIndex : Outport  Port=2
  wires:
  Constant/1 -> Switch Case Action Subsystem/1(In1)
  Case/1 -> Switch Case Action Subsystem/Action
  Switch Case Action Subsystem/1(Out1) -> Merge/1
  Merge/1 -> Enable/1
  Case Default/1 -> Switch Case Action Subsystem1/Action
  Constant1/1 -> Switch Case Action Subsystem1/1(In1)
  Switch Case Action Subsystem1/1(Default) -> Merge/2
  Constant2/1 -> FinishIndex/1

== system Robot/Motor2 Torque Control Init Frame/State_8_Enable/Subsystem ==
  Case : Inport
  Case Default : Inport  Port=2
  Constant : Constant
  Constant1 : Constant  Value=0
  Constant2 : Constant  Value=TaskIndex
  Merge : Merge
  Switch Case Action Subsystem : Subsystem  TreatAsAtomicUnit=on
  Switch Case Action Subsystem1 : Subsystem  TreatAsAtomicUnit=on
  Enable : Outport
  FinishIndex : Outport  Port=2
  wires:
  Constant/1 -> Switch Case Action Subsystem/1(In1)
  Case/1 -> Switch Case Action Subsystem/Action
  Switch Case Action Subsystem/1(Out1) -> Merge/1
  Merge/1 -> Enable/1
  Case Default/1 -> Switch Case Action Subsystem1/Action
  Constant1/1 -> Switch Case Action Subsystem1/1(In1)
  Switch Case Action Subsystem1/1(Default) -> Merge/2
  Constant2/1 -> FinishIndex/1

== system Robot/Motor2 Torque Control Init Frame/State_9_Enable/Subsystem ==
  Case : Inport
  Case Default : Inport  Port=2
  Constant : Constant
  Constant1 : Constant  Value=0
  Constant2 : Constant  Value=TaskIndex
  Merge : Merge
  Switch Case Action Subsystem : Subsystem  TreatAsAtomicUnit=on
  Switch Case Action Subsystem1 : Subsystem  TreatAsAtomicUnit=on
  Enable : Outport
  FinishIndex : Outport  Port=2
  wires:
  Constant/1 -> Switch Case Action Subsystem/1(In1)
  Case/1 -> Switch Case Action Subsystem/Action
  Switch Case Action Subsystem/1(Out1) -> Merge/1
  Merge/1 -> Enable/1
  Case Default/1 -> Switch Case Action Subsystem1/Action
  Constant1/1 -> Switch Case Action Subsystem1/1(In1)
  Switch Case Action Subsystem1/1(Default) -> Merge/2
  Constant2/1 -> FinishIndex/1

== system Robot/Motor3 Torque Control Init Frame/Get MasterState OP Frame/If Action Subsystem5 ==
  In1 : Inport
  Action Port : ActionPort  ActionPortLabel=if((u1 == 8))
  Out1 : Outport
  wires:
  In1/1 -> Out1/1

== system Robot/Motor3 Torque Control Init Frame/Get MasterState OP Frame/If Action Subsystem6 ==
  In1 : Inport
  Action Port : ActionPort  ActionPortLabel=else
  Out1 : Outport
  wires:
  In1/1 -> Out1/1

== system Robot/Motor3 Torque Control Init Frame/Get MasterState OP Frame/If Action Subsystem7 ==
  In1 : Inport
  Action Port : ActionPort  ActionPortLabel=if((u1 == 4663))
  Discrete-Time Integrator : DiscreteIntegrator  SampleTime=-1  ICPrevOutput=DiscIntNeverNeededParam  ICPrevScaledInput=DiscIntNeverNeededParam
  Out1 : Outport
  wires:
  In1/1 -> Discrete-Time Integrator/1
  Discrete-Time Integrator/1 -> Out1/1

== system Robot/Motor3 Torque Control Init Frame/PDO Set 0x6040:6->7->15 Frame/If Action Subsystem ==
  In1 : Inport
  Action Port : ActionPort  ActionPortLabel=if((u1 == 720)&(u2 == 500))
  Out1 : Outport
  wires:
  In1/1 -> Out1/1

== system Robot/Motor3 Torque Control Init Frame/PDO Set 0x6040:6->7->15 Frame/If Action Subsystem1 ==
  In1 : Inport
  Action Port : ActionPort  ActionPortLabel=elseif((u1 == 689)&(u2 == 500))
  Out1 : Outport
  wires:
  In1/1 -> Out1/1

== system Robot/Motor3 Torque Control Init Frame/PDO Set 0x6040:6->7->15 Frame/If Action Subsystem2 ==
  In1 : Inport
  Action Port : ActionPort  ActionPortLabel=elseif( (u1 == 691)&(u2 == 500))
  Out1 : Outport
  wires:
  In1/1 -> Out1/1

== system Robot/Motor3 Torque Control Init Frame/PDO Set 0x6040:6->7->15 Frame/If Action Subsystem4 ==
  In1 : Inport
  Action Port : ActionPort  ActionPortLabel=else
  Out1 : Outport
  wires:
  In1/1 -> Out1/1

== system Robot/Motor3 Torque Control Init Frame/PDO Set 0x6040:6->7->15 Frame/If Action Subsystem5 ==
  In1 : Inport
  Action Port : ActionPort  ActionPortLabel=if((u1 >= 0.1))
  Out1 : Outport
  wires:
  In1/1 -> Out1/1

== system Robot/Motor3 Torque Control Init Frame/PDO Set 0x6040:6->7->15 Frame/If Action Subsystem6 ==
  In1 : Inport
  Action Port : ActionPort  ActionPortLabel=else
  Out1 : Outport
  wires:
  In1/1 -> Out1/1

== system Robot/Motor3 Torque Control Init Frame/PDO Set 0x6040:6->7->15 Frame/If Action Subsystem7 ==
  In1 : Inport
  Action Port : ActionPort  ActionPortLabel=if((u1 == 4663)|(u1 == 4791))
  Discrete-Time Integrator : DiscreteIntegrator  SampleTime=-1  ICPrevOutput=DiscIntNeverNeededParam  ICPrevScaledInput=DiscIntNeverNeededParam
  Out1 : Outport
  wires:
  In1/1 -> Discrete-Time Integrator/1
  Discrete-Time Integrator/1 -> Out1/1

== system Robot/Motor3 Torque Control Init Frame/SDO Get 0x6075 Frame/If Action Subsystem5 ==
  In1 : Inport
  Action Port : ActionPort  ActionPortLabel=if((u1 == 2))
  Out1 : Outport
  wires:
  In1/1 -> Out1/1

== system Robot/Motor3 Torque Control Init Frame/SDO Get 0x6075 Frame/If Action Subsystem6 ==
  In1 : Inport
  Action Port : ActionPort  ActionPortLabel=else
  Out1 : Outport
  wires:
  In1/1 -> Out1/1

== system Robot/Motor3 Torque Control Init Frame/SDO Get 0x6075 Frame/If Action Subsystem7 ==
  In1 : Inport
  Action Port : ActionPort  ActionPortLabel=if((u1 == 4663))
  Discrete-Time Integrator : DiscreteIntegrator  SampleTime=-1  ICPrevOutput=DiscIntNeverNeededParam  ICPrevScaledInput=DiscIntNeverNeededParam
  Out1 : Outport
  wires:
  In1/1 -> Discrete-Time Integrator/1
  Discrete-Time Integrator/1 -> Out1/1

== system Robot/Motor3 Torque Control Init Frame/SDO Set 0x6040:15 Frame/If Action Subsystem1 ==
  In1 : Inport
  Action Port : ActionPort
  Out1 : Outport
  wires:
  In1/1 -> Out1/1

== system Robot/Motor3 Torque Control Init Frame/SDO Set 0x6040:15 Frame/If Action Subsystem2 ==
  In1 : Inport
  Action Port : ActionPort
  Out1 : Outport
  wires:
  In1/1 -> Out1/1

== system Robot/Motor3 Torque Control Init Frame/SDO Set 0x6040:15 Frame/If Action Subsystem3 ==
  In1 : Inport
  Action Port : ActionPort
  Discrete-Time Integrator : DiscreteIntegrator  SampleTime=-1  ICPrevOutput=DiscIntNeverNeededParam  ICPrevScaledInput=DiscIntNeverNeededParam
  Out1 : Outport
  wires:
  In1/1 -> Discrete-Time Integrator/1
  Discrete-Time Integrator/1 -> Out1/1

== system Robot/Motor3 Torque Control Init Frame/SDO Set 0x6040:15 Frame/If Action Subsystem5 ==
  In1 : Inport
  Action Port : ActionPort
  Out1 : Outport
  wires:
  In1/1 -> Out1/1

== system Robot/Motor3 Torque Control Init Frame/SDO Set 0x6040:15 Frame/If Action Subsystem6 ==
  In1 : Inport
  Action Port : ActionPort
  Out1 : Outport
  wires:
  In1/1 -> Out1/1

== system Robot/Motor3 Torque Control Init Frame/SDO Set 0x6040:15 Frame/If Action Subsystem7 ==
  In1 : Inport
  Action Port : ActionPort
  Discrete-Time Integrator : DiscreteIntegrator  SampleTime=-1  ICPrevOutput=DiscIntNeverNeededParam  ICPrevScaledInput=DiscIntNeverNeededParam
  Out1 : Outport
  wires:
  In1/1 -> Discrete-Time Integrator/1
  Discrete-Time Integrator/1 -> Out1/1

== system Robot/Motor3 Torque Control Init Frame/SDO Set 0x6040:31 Frame/If Action Subsystem1 ==
  In1 : Inport
  Action Port : ActionPort
  Out1 : Outport
  wires:
  In1/1 -> Out1/1

== system Robot/Motor3 Torque Control Init Frame/SDO Set 0x6040:31 Frame/If Action Subsystem2 ==
  In1 : Inport
  Action Port : ActionPort
  Out1 : Outport
  wires:
  In1/1 -> Out1/1

== system Robot/Motor3 Torque Control Init Frame/SDO Set 0x6040:31 Frame/If Action Subsystem3 ==
  In1 : Inport
  Action Port : ActionPort
  Discrete-Time Integrator : DiscreteIntegrator  SampleTime=-1  ICPrevOutput=DiscIntNeverNeededParam  ICPrevScaledInput=DiscIntNeverNeededParam
  Out1 : Outport
  wires:
  In1/1 -> Discrete-Time Integrator/1
  Discrete-Time Integrator/1 -> Out1/1

== system Robot/Motor3 Torque Control Init Frame/SDO Set 0x6040:31 Frame/If Action Subsystem5 ==
  In1 : Inport
  Action Port : ActionPort
  Out1 : Outport
  wires:
  In1/1 -> Out1/1

== system Robot/Motor3 Torque Control Init Frame/SDO Set 0x6040:31 Frame/If Action Subsystem6 ==
  In1 : Inport
  Action Port : ActionPort
  Out1 : Outport
  wires:
  In1/1 -> Out1/1

== system Robot/Motor3 Torque Control Init Frame/SDO Set 0x6040:31 Frame/If Action Subsystem7 ==
  In1 : Inport
  Action Port : ActionPort
  Discrete-Time Integrator : DiscreteIntegrator  SampleTime=-1  ICPrevOutput=DiscIntNeverNeededParam  ICPrevScaledInput=DiscIntNeverNeededParam
  Out1 : Outport
  wires:
  In1/1 -> Discrete-Time Integrator/1
  Discrete-Time Integrator/1 -> Out1/1

== system Robot/Motor3 Torque Control Init Frame/SDO Set 0x6040:6 Frame/If Action Subsystem1 ==
  In1 : Inport
  Action Port : ActionPort
  Out1 : Outport
  wires:
  In1/1 -> Out1/1

== system Robot/Motor3 Torque Control Init Frame/SDO Set 0x6040:6 Frame/If Action Subsystem2 ==
  In1 : Inport
  Action Port : ActionPort
  Out1 : Outport
  wires:
  In1/1 -> Out1/1

== system Robot/Motor3 Torque Control Init Frame/SDO Set 0x6040:6 Frame/If Action Subsystem3 ==
  In1 : Inport
  Action Port : ActionPort
  Discrete-Time Integrator : DiscreteIntegrator  SampleTime=-1  ICPrevOutput=DiscIntNeverNeededParam  ICPrevScaledInput=DiscIntNeverNeededParam
  Out1 : Outport
  wires:
  In1/1 -> Discrete-Time Integrator/1
  Discrete-Time Integrator/1 -> Out1/1

== system Robot/Motor3 Torque Control Init Frame/SDO Set 0x6040:6 Frame/If Action Subsystem5 ==
  In1 : Inport
  Action Port : ActionPort
  Out1 : Outport
  wires:
  In1/1 -> Out1/1

== system Robot/Motor3 Torque Control Init Frame/SDO Set 0x6040:6 Frame/If Action Subsystem6 ==
  In1 : Inport
  Action Port : ActionPort
  Out1 : Outport
  wires:
  In1/1 -> Out1/1

== system Robot/Motor3 Torque Control Init Frame/SDO Set 0x6040:6 Frame/If Action Subsystem7 ==
  In1 : Inport
  Action Port : ActionPort
  Discrete-Time Integrator : DiscreteIntegrator  SampleTime=-1  ICPrevOutput=DiscIntNeverNeededParam  ICPrevScaledInput=DiscIntNeverNeededParam
  Out1 : Outport
  wires:
  In1/1 -> Discrete-Time Integrator/1
  Discrete-Time Integrator/1 -> Out1/1

== system Robot/Motor3 Torque Control Init Frame/SDO Set 0x6040:7 Frame/If Action Subsystem1 ==
  In1 : Inport
  Action Port : ActionPort
  Out1 : Outport
  wires:
  In1/1 -> Out1/1

== system Robot/Motor3 Torque Control Init Frame/SDO Set 0x6040:7 Frame/If Action Subsystem2 ==
  In1 : Inport
  Action Port : ActionPort
  Out1 : Outport
  wires:
  In1/1 -> Out1/1

== system Robot/Motor3 Torque Control Init Frame/SDO Set 0x6040:7 Frame/If Action Subsystem3 ==
  In1 : Inport
  Action Port : ActionPort
  Discrete-Time Integrator : DiscreteIntegrator  SampleTime=-1  ICPrevOutput=DiscIntNeverNeededParam  ICPrevScaledInput=DiscIntNeverNeededParam
  Out1 : Outport
  wires:
  In1/1 -> Discrete-Time Integrator/1
  Discrete-Time Integrator/1 -> Out1/1

== system Robot/Motor3 Torque Control Init Frame/SDO Set 0x6040:7 Frame/If Action Subsystem5 ==
  In1 : Inport
  Action Port : ActionPort
  Out1 : Outport
  wires:
  In1/1 -> Out1/1

== system Robot/Motor3 Torque Control Init Frame/SDO Set 0x6040:7 Frame/If Action Subsystem6 ==
  In1 : Inport
  Action Port : ActionPort
  Out1 : Outport
  wires:
  In1/1 -> Out1/1

== system Robot/Motor3 Torque Control Init Frame/SDO Set 0x6040:7 Frame/If Action Subsystem7 ==
  In1 : Inport
  Action Port : ActionPort
  Discrete-Time Integrator : DiscreteIntegrator  SampleTime=-1  ICPrevOutput=DiscIntNeverNeededParam  ICPrevScaledInput=DiscIntNeverNeededParam
  Out1 : Outport
  wires:
  In1/1 -> Discrete-Time Integrator/1
  Discrete-Time Integrator/1 -> Out1/1

== system Robot/Motor3 Torque Control Init Frame/SDO Set 0x6060:10 Frame/If Action Subsystem5 ==
  In1 : Inport
  Action Port : ActionPort  ActionPortLabel=if((u1 == 2))
  Out1 : Outport
  wires:
  In1/1 -> Out1/1

== system Robot/Motor3 Torque Control Init Frame/SDO Set 0x6060:10 Frame/If Action Subsystem6 ==
  In1 : Inport
  Action Port : ActionPort  ActionPortLabel=else
  Out1 : Outport
  wires:
  In1/1 -> Out1/1

== system Robot/Motor3 Torque Control Init Frame/SDO Set 0x6060:10 Frame/If Action Subsystem7 ==
  In1 : Inport
  Action Port : ActionPort  ActionPortLabel=if((u1 == 4663))
  Discrete-Time Integrator : DiscreteIntegrator  SampleTime=-1  ICPrevOutput=DiscIntNeverNeededParam  ICPrevScaledInput=DiscIntNeverNeededParam
  Out1 : Outport
  wires:
  In1/1 -> Discrete-Time Integrator/1
  Discrete-Time Integrator/1 -> Out1/1

== system Robot/Motor3 Torque Control Init Frame/SDO Set 0x6060:6 Frame/If Action Subsystem5 ==
  In1 : Inport
  Action Port : ActionPort
  Out1 : Outport
  wires:
  In1/1 -> Out1/1

== system Robot/Motor3 Torque Control Init Frame/SDO Set 0x6060:6 Frame/If Action Subsystem6 ==
  In1 : Inport
  Action Port : ActionPort
  Out1 : Outport
  wires:
  In1/1 -> Out1/1

== system Robot/Motor3 Torque Control Init Frame/SDO Set 0x6060:6 Frame/If Action Subsystem7 ==
  In1 : Inport
  Action Port : ActionPort
  Discrete-Time Integrator : DiscreteIntegrator  SampleTime=-1  ICPrevOutput=DiscIntNeverNeededParam  ICPrevScaledInput=DiscIntNeverNeededParam
  Out1 : Outport
  wires:
  In1/1 -> Discrete-Time Integrator/1
  Discrete-Time Integrator/1 -> Out1/1

== system Robot/Motor3 Torque Control Init Frame/SDO Set 0x6080:-1 Frame/If Action Subsystem5 ==
  In1 : Inport
  Action Port : ActionPort  ActionPortLabel=if((u1 == 2))
  Out1 : Outport
  wires:
  In1/1 -> Out1/1

== system Robot/Motor3 Torque Control Init Frame/SDO Set 0x6080:-1 Frame/If Action Subsystem6 ==
  In1 : Inport
  Action Port : ActionPort  ActionPortLabel=else
  Out1 : Outport
  wires:
  In1/1 -> Out1/1

== system Robot/Motor3 Torque Control Init Frame/SDO Set 0x6080:-1 Frame/If Action Subsystem7 ==
  In1 : Inport
  Action Port : ActionPort  ActionPortLabel=if((u1 == 4663))
  Discrete-Time Integrator : DiscreteIntegrator  SampleTime=-1  ICPrevOutput=DiscIntNeverNeededParam  ICPrevScaledInput=DiscIntNeverNeededParam
  Out1 : Outport
  wires:
  In1/1 -> Discrete-Time Integrator/1
  Discrete-Time Integrator/1 -> Out1/1

== system Robot/Motor3 Torque Control Init Frame/SDO Set 0x6098:35 Frame/If Action Subsystem5 ==
  In1 : Inport
  Action Port : ActionPort
  Out1 : Outport
  wires:
  In1/1 -> Out1/1
